simulink model "test"  (Simulink 7.1)
settings: Solver=ode15s  StartTime=0.0  StopTime=10  MaxStep=0.2  RelTol=1e-3
libraries: fl_lib x9, nesl_utility x6, sh_lib x4
settings Model: Creator=Cmo  LastModifiedBy=Cmo
settings OptimizationCC: BlockReduction=off

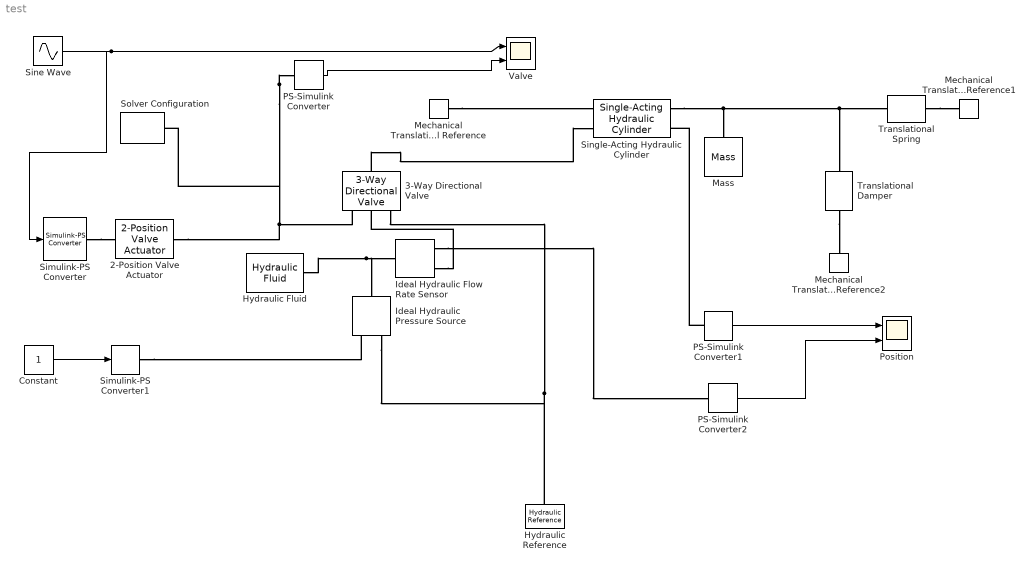
== system test ==
  2-Position Valve Actuator : sh_lib/Valves/Valve Actuators/2-Position Valve Actuator  DialogController=NetworkEngine.DynNeDlgSource  SystemSampleTime=-1  stroke=0.01 m  t_on=0.1 s  t_off=0.1 s  act_signal=24  init_position=0  act_orientation=1  LocalVarLogging=[]
  3-Way Directional Valve : sh_lib/Valves/Directional Valves/3-Way Directional Valve  Orientation=down  DialogController=NetworkEngine.DynNeDlgSource  SystemSampleTime=-1  mdl_type=1  area_max=1e-4 m^2  opening_max=0.01 m  opening_tab="[  -0.002 0 0.002 0.005 0.015 ] m"  area_tab="[  1e-09 2.0352e-07 4.0736e-05 0.00011438 0.00034356 ] m^2"  pressure_tab="[  -1e+07 -5e+06 -2e+06 2e+06 5e+06 1e+07 ] Pa"  flow_rate_tab="[  -1e-07 -7.0711e-08 -4.4721e-08 4.4721e-08 7.0711e-08 1e-07 ; -2.0352e-05 -1.4391e-05 -9.1017e-06 9.1017e-06 1.4391e-05 2.0352e-05 ; -0.0040736 -0.0028805 -0.0018218 0.0018218 0.0028805 0.0040736 ; -0.011438 -0.0080879 -0.0051152 0.0051152 0.0080879 0.011438 ; -0.034356 -0.024293 -0.015364 0.015364 0.024293 0.034356 ; ] m^3/s"  interp_method=1  extrap_method=1  C_d=0.7  x_0_P=0 m  x_0_T=0.08 m  Re_cr=12  A_leak=1e-6 m^2  LocalVarLogging=[]
  Constant : Constant  OutDataType=sfix(16)  OutScaling=2^0
  Hydraulic Fluid : sh_lib/Hydraulic Utilities/Hydraulic Fluid  DialogController=NetworkEngine.DynNeDlgSource  SystemSampleTime=-1  DataSource=1  SelFluid=3  SysTemp=40 c  TrapAir=0.002  ViscDerFactor=1  LocalVarLogging=[]
  Hydraulic Reference : fl_lib/Hydraulic/Hydraulic Elements/Hydraulic Reference  Orientation=down  DialogController=NetworkEngine.DynNeDlgSource  SystemSampleTime=-1  LocalVarLogging=[]
  Ideal Hydraulic Pressure Source : fl_lib/Hydraulic/Hydraulic Sensors and Sources/Ideal Hydraulic Pressure Source  Orientation=down  DialogController=NetworkEngine.DynNeDlgSource  SystemSampleTime=-1  flow_rate_Log=off  pr_differential_Log=off  power_Log=off  LocalVarNames=|flow_rate|pr_differential|power  LocalVarDescs=|Flow rate through the source (m^3/s)|Pressure differential across the source (Pa)|Source power (W)  LocalVarLogging=[0 0 0]
  Ideal Hydraulic Flow Rate Sensor : fl_lib/Hydraulic/Hydraulic Sensors and Sources/Ideal Hydraulic Flow Rate Sensor  DialogController=NetworkEngine.DynNeDlgSource  SystemSampleTime=-1  LocalVarLogging=[]
  Mass : fl_lib/Mechanical/Translational Elements/Mass  Orientation=down  DialogController=NetworkEngine.DynNeDlgSource  SystemSampleTime=-1  mass=5 kg  initial_velocity=0 m/s  force_Log=off  velocity_Log=off  LocalVarNames=|force|velocity  LocalVarDescs=|Inertia force (N)|Mass absolute velocity (m/s)  LocalVarLogging=[0 0]
  Mechanical Translational Reference : fl_lib/Mechanical/Translational Elements/Mechanical Translational Reference  Orientation=left  DialogController=NetworkEngine.DynNeDlgSource  SystemSampleTime=-1  LocalVarLogging=[]
  Mechanical Translational Reference1 : fl_lib/Mechanical/Translational Elements/Mechanical Translational Reference  DialogController=NetworkEngine.DynNeDlgSource  SystemSampleTime=-1  LocalVarLogging=[]
  Mechanical Translational Reference2 : fl_lib/Mechanical/Translational Elements/Mechanical Translational Reference  Orientation=down  DialogController=NetworkEngine.DynNeDlgSource  SystemSampleTime=-1  LocalVarLogging=[]
  PS-Simulink Converter : nesl_utility/PS-Simulink Converter  DialogController=NetworkEngine.DynNeUtilDlgSource  SystemSampleTime=-1  PhysicalDomain=network_engine_domain  LeftPortType=input  RightPortType=output  SubClassName=ps_output  Unit=1  AffineConversion=off
  PS-Simulink Converter1 : nesl_utility/PS-Simulink Converter  DialogController=NetworkEngine.DynNeUtilDlgSource  SystemSampleTime=-1  PhysicalDomain=network_engine_domain  LeftPortType=input  RightPortType=output  SubClassName=ps_output  Unit=1  AffineConversion=off
  PS-Simulink Converter2 : nesl_utility/PS-Simulink Converter  DialogController=NetworkEngine.DynNeUtilDlgSource  SystemSampleTime=-1  PhysicalDomain=network_engine_domain  LeftPortType=input  RightPortType=output  SubClassName=ps_output  Unit=1  AffineConversion=off
  Position : Scope  NumInputPorts=2
      settings: YMin=-0.0004~-5  YMax=0~5
  Simulink-PS Converter : nesl_utility/Simulink-PS Converter  DialogController=NetworkEngine.DynNeUtilDlgSource  SystemSampleTime=-1  PhysicalDomain=network_engine_domain  LeftPortType=input  RightPortType=output  SubClassName=ps_input  Unit=1  AffineConversion=off
  Simulink-PS Converter1 : nesl_utility/Simulink-PS Converter  DialogController=NetworkEngine.DynNeUtilDlgSource  SystemSampleTime=-1  PhysicalDomain=network_engine_domain  LeftPortType=input  RightPortType=output  SubClassName=ps_input  Unit=1  AffineConversion=off
  Sine Wave : Sin  Amplitude=50  SampleTime=0
  Single-Acting Hydraulic Cylinder : sh_lib/Hydraulic Cylinders/Single-Acting Hydraulic Cylinder  DialogController=NetworkEngine.DynNeDlgSource  SystemSampleTime=-1  area=0.002 m^2  stroke=0.25 m  init_pos=0.05 m  dead_vol=1e-06 m^3  k_sh=1.4  stiff=1e+07 N/m  D=250 N/(m/s)  or=1  LocalVarLogging=[]
  Solver Configuration : nesl_utility/Solver Configuration  DialogController=NetworkEngine.DynNeUtilDlgSource  SystemSampleTime=-1  PhysicalDomain=network_engine_domain  LeftPortType=input  RightPortType=generic  SubClassName=solver  Accelerate=off  Profile=off  ResidualTolerance=1e-9  MaxNonlinIter=12  MaxModeIter=2  DoFixedCost=off  DoDC=off  LinearAlgebra=Sparse
  Translational Damper : fl_lib/Mechanical/Translational Elements/Translational Damper  Orientation=down  DialogController=NetworkEngine.DynNeDlgSource  SystemSampleTime=-1  D=250 N/(m/s)  force_Log=off  rel_velocity_Log=off  power_Log=off  LocalVarNames=|force|rel_velocity|power  LocalVarDescs=|Damping force (N)|Damper relative velocity (m/s)|Power dissipated in the damper (W)  LocalVarLogging=[0 0 0]
  Translational Spring : fl_lib/Mechanical/Translational Elements/Translational Spring  DialogController=NetworkEngine.DynNeDlgSource  SystemSampleTime=-1  spr_rate=6e3 N/m  init_def=0.2 m  force_Log=off  deformation_Log=off  LocalVarNames=|force|deformation  LocalVarDescs=|Spring force (N)|Spring deformation (m)  LocalVarLogging=[0 0]
  Valve : Scope  NumInputPorts=2
      settings: TimeRange=10  YMin=-20~0  YMax=20~0.01
  wires:
  Sine Wave/1 -> Simulink-PS Converter/1, Valve/1
  PS-Simulink Converter/1 -> Valve/2
  PS-Simulink Converter1/1 -> Position/1
  Constant/1 -> Simulink-PS Converter1/1
  PS-Simulink Converter2/1 -> Position/2
  connections:
  Hydraulic Reference/LConn1 -- 3-Way Directional Valve/RConn3 -- Ideal Hydraulic Pressure Source/RConn2
  Hydraulic Fluid/RConn1 -- Ideal Hydraulic Pressure Source/LConn1 -- Ideal Hydraulic Flow Rate Sensor/LConn1
  Mechanical Translational Reference/LConn1 -- Single-Acting Hydraulic Cylinder/LConn1
  Translational Spring/RConn1 -- Mechanical Translational Reference1/LConn1
  Translational Damper/RConn1 -- Mechanical Translational Reference2/LConn1
  Single-Acting Hydraulic Cylinder/RConn1 -- Translational Spring/LConn1 -- Translational Damper/LConn1 -- Mass/LConn1
  PS-Simulink Converter/LConn1 -- Solver Configuration/RConn1 -- 3-Way Directional Valve/RConn1 -- 2-Position Valve Actuator/RConn1
  Simulink-PS Converter/RConn1 -- 2-Position Valve Actuator/LConn1
  Simulink-PS Converter1/RConn1 -- Ideal Hydraulic Pressure Source/RConn1
  PS-Simulink Converter1/LConn1 -- Single-Acting Hydraulic Cylinder/RConn2
  Ideal Hydraulic Flow Rate Sensor/RConn1 -- PS-Simulink Converter2/LConn1
  3-Way Directional Valve/LConn1 -- Single-Acting Hydraulic Cylinder/LConn2
  Ideal Hydraulic Flow Rate Sensor/RConn2 -- 3-Way Directional Valve/RConn2
